simulink model "test"  (R2019a)
settings: Solver=VariableStepAuto  StartTime=0.0  StopTime=10  RelTol=1e-3
settings Model: Creator=Lenovo  LastModifiedBy=Lenovo
settings DataIOCC: SaveFormat=Array  SaveState=on

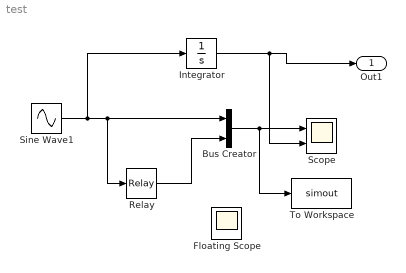
== system test ==
  Bus Creator : BusCreator  Inputs=2
  Floating Scope : Scope
      settings: Floating=on
  Integrator : Integrator
  Relay : Relay  OffOutputValue=-1
  Scope : Scope  NumInputPorts=2
  Sine Wave1 : Sin  SampleTime=0
  To Workspace : ToWorkspace  VariableName=simout  SaveFormat=Timeseries  SampleTime=-1
  Out1 : Outport
  wires:
  Sine Wave1/1 -> Integrator/1, Relay/1, Bus Creator/1
  Relay/1 -> Bus Creator/2
  Bus Creator/1 -> To Workspace/1, Scope/1
  Integrator/1 -> Scope/2, Out1/1
